simulink model "Autovalores_Reales"  (R2014a)
settings: Solver=ode45  StartTime=0.0  StopTime=10.0  RelTol=1e-3
values from neighbouring files (symbols this model uses):
  Ci1 = 0.5    [Autovalores_Reales_Parametros.m]    (also in Masa_Resorte_Duro_Parametros.m = 0)
  Ci2 = 0.5    [Autovalores_Reales_Parametros.m]    (also in Masa_Resorte_Duro_Parametros.m = 0)
  L1 = -1    [Autovalores_Reales_Parametros.m]
  L2 = -2    [Autovalores_Reales_Parametros.m]
libraries: simulink x1
settings Model: Creator=Jose  LastModifiedBy=Jose

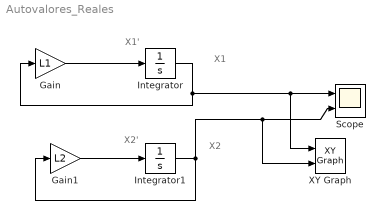
== system Autovalores_Reales ==
  note: X2
  note: X1
  note: X2'
  note: X1'
  Gain : Gain  Gain=L1
  Gain1 : Gain  Gain=L2
  Integrator : Integrator  InitialCondition=Ci1
  Integrator1 : Integrator  InitialCondition=Ci2
  Scope : Scope  NumInputPorts=2
      settings: YMin=-5~-5  YMax=5~5
  XY Graph : simulink/Sinks/XY Graph  xmin=-1  xmax=1  ymin=-1  ymax=1  st=-1
  wires:
  Integrator/1 -> XY Graph/1, Scope/1, Gain/1
  Gain/1 -> Integrator/1
  Integrator1/1 -> Gain1/1, XY Graph/2, Scope/2
  Gain1/1 -> Integrator1/1
